simulink model "watertank"  (Simulink 5.0)
settings: Solver=ode45  StartTime=0.0  StopTime=200.0  RelTol=1e-3
PreLoadFcn:
  | watertankdat
values from neighbouring files (symbols this model uses):
  a = 2    [watertankdat.m]
  A = 20    [watertankdat.m]
  b = 5    [watertankdat.m]
settings Model: Creator=lparsons  LastModifiedBy=lparsons  SignalLoggingName=logsOut  ZeroCrossControl=UseLocalSettings  TargetHWChar=2  TargetHWWordLengths=8,16,32,32  RTWMathFcnLibMatFile=iso_c_tmw.mat  RTWOptions="-aEnforceIntegerDowncast=1 -aFoldNonRolledExpr=1 -aInlineInvariantSignals=1 -aInlineParameters=0 -aLocalBlockOutputs=1 -aRollThreshold=5 -aGenerateReport=0 -aGenCodeOnly=0 -aRTWVerbose=1 -aForceParamTrailComments=0 -aGenerateComments=1 -aIgnoreCustomStorageClasses=1 -aIncHierarchyInIds=0 -aMaxRTWIdLen=31 -aShowEliminatedStatements=0 -aPrefixModelToSubsysFcnNames=1 -aIncDataTypeInIds=0 -aInlinedPrmAccess=\"Literals\" -aTargetFcnLib=\"iso_c_tmw.mat\" -aGenerateFullHeader=1 -aIsPILTarget=0 -aExtMode=0 -aExtModeStaticAlloc=0 -aExtModeTesting=0 -aExtModeStaticAllocSize=1000000 -aExtModeTransport=0 -aLogVarNameModifier=\"rt_\" -aRTWCAPISignals=0 -aRTWCAPIParams=0 -aDialogCategory=0"
settings DataIOCC: LimitDataPoints=on  SaveFormat=Array  SignalLoggingName=logsOut
settings OptimizationCC: InlineInvariantSignals=on  MultiInstanced=off
settings FormatCC: IgnoreBidirectionalLines=off  ExecutionOrder=off
settings HardwareCC: ProdHWDeviceType=Microprocessor  ShiftRightIntArith=on  TargetHWCharacteristics=InheritFromRTWHook  ProdIntDivRoundTo=Undefined
settings CodeAppCC: FileBanners=off
settings GRTTargetCC: TargetFcnLib=iso_c_tmw.mat  IsERTTarget=off

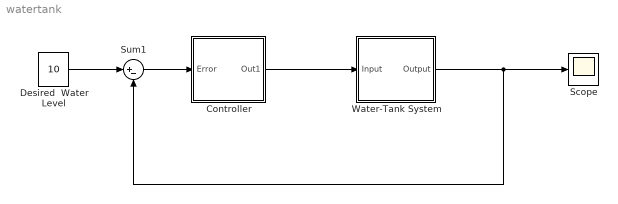
== system watertank ==
  Controller : Subsystem
  Desired  Water Level : Constant  Value=10
  Scope : Scope
  Sum1 : Sum  Inputs=|+-  SaturateOnIntegerOverflow=on
  Water-Tank System : Subsystem
  wires:
  Desired  Water Level/1 -> Sum1/1
  Sum1/1 -> Controller/1(Error)
  Water-Tank System/1(Output) -> Sum1/2, Scope/1
  Controller/1(Out1) -> Water-Tank System/1(Input)

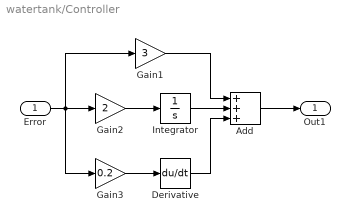
== system watertank/Controller ==
  Error : Inport
  Add : Sum  Inputs=+++  OutScaling=2^-10
  Derivative : Derivative
  Gain1 : Gain  Gain=3  SaturateOnIntegerOverflow=on
  Gain2 : Gain  Gain=2  SaturateOnIntegerOverflow=on
  Gain3 : Gain  Gain=0.2  SaturateOnIntegerOverflow=on
  Integrator : Integrator
  Out1 : Outport
  wires:
  Error/1 -> Gain2/1, Gain1/1, Gain3/1
  Gain2/1 -> Integrator/1
  Integrator/1 -> Add/2
  Add/1 -> Out1/1
  Gain1/1 -> Add/1
  Gain3/1 -> Derivative/1
  Derivative/1 -> Add/3

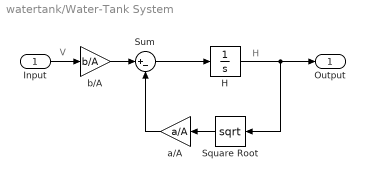
== system watertank/Water-Tank System ==
  note: H
  note: V
  Input : Inport
  H : Integrator
  Square Root : Math  Orientation=left  Operator=sqrt  OutputSignalType=real
  Sum : Sum  Inputs=|+-  SaturateOnIntegerOverflow=on
  a/A : Gain  Orientation=left  Gain=a/A  SaturateOnIntegerOverflow=on
  b/A : Gain  Gain=b/A  SaturateOnIntegerOverflow=on
  Output : Outport
  wires:
  b/A/1 -> Sum/1
  Sum/1 -> H/1
  H/1 -> Square Root/1, Output/1
  Square Root/1 -> a/A/1
  a/A/1 -> Sum/2
  Input/1 -> b/A/1
